simulink model "quad_LQRwithIntegrators_sim"  (R2020a)
settings: Solver=ode4  StartTime=0.0  StopTime=5  FixedStep=0.001  RelTol=1e-3
values from neighbouring files (symbols this model uses):
  L = 0.2    [anim_2Dquad.m]    (also in anim_2Dquad_intercept.m)
undefined symbols (not defined in the file or in its folder): g, I, K_aug, m
settings Model: Creator=Amir  LastModifiedBy=alex
settings DataIOCC: ReturnWorkspaceOutputs=off
settings DebuggingCC: ArithmeticOperatorsInVariantConditions=warning
settings SFSimCC: CustomCodeUndefinedFunction=UseInterfaceOnly

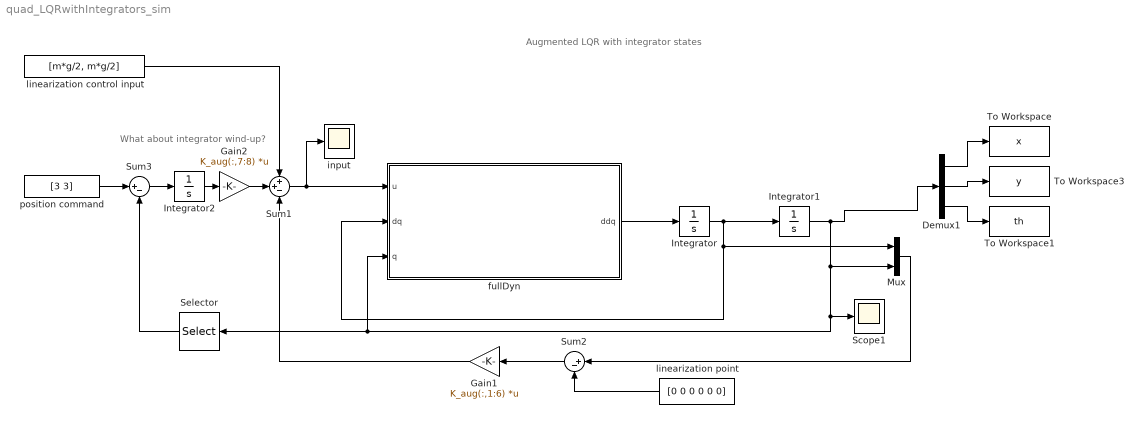
== system quad_LQRwithIntegrators_sim ==
  note: Augmented LQR with integrator states
  note: What about integrator wind-up?
  Demux1 : Demux  Outputs=3
  Gain1 : Gain  Gain=K_aug(:,1:6)  Multiplication=Matrix(K*u)
  Gain2 : Gain  Gain=K_aug(:,7:8)  Multiplication=Matrix(K*u)
  Integrator : Integrator  InitialCondition=[0 0 0]
  Integrator1 : Integrator  InitialCondition=[0, 0, 0]
  Integrator2 : Integrator
  Mux : Mux  Inputs=2
  Scope1 : Scope
  Selector : Selector  InputPortWidth=3  IndexOptions=Index vector (dialog)  Indices=[1 2]  OutputSizes=1
  Sum1 : Sum  Inputs=++-
  Sum2 : Sum  Inputs=|+-
  Sum3 : Sum  Inputs=|+-
  To Workspace : ToWorkspace  VariableName=x  SaveFormat=Structure With Time  SampleTime=0.01
  To Workspace1 : ToWorkspace  VariableName=th  SaveFormat=Structure With Time  SampleTime=0.01
  To Workspace3 : ToWorkspace  VariableName=y  SaveFormat=Structure With Time  SampleTime=0.01
  fullDyn : MATLAB Function  TreatAsAtomicUnit=on
  input : Scope
  linearization control input : Constant  Value=[m*g/2, m*g/2]
  linearization point : Constant  Value=[0 0 0 0 0 0]
  position command : Constant  Value=[3 3]
  wires:
  fullDyn/1(ddq) -> Integrator/1
  Integrator/1 -> Integrator1/1, Mux/1, fullDyn/2(dq)
  Integrator1/1 -> Demux1/1, Mux/2, Scope1/1, fullDyn/3(q), Selector/1
  Sum1/1 -> input/1, fullDyn/1(u)
  Sum2/1 -> Gain1/1
  linearization point/1 -> Sum2/2
  Mux/1 -> Sum2/1
  linearization control input/1 -> Sum1/1
  Gain1/1 -> Sum1/3
  Integrator2/1 -> Gain2/1
  Gain2/1 -> Sum1/2
  Sum3/1 -> Integrator2/1
  position command/1 -> Sum3/1
  Selector/1 -> Sum3/2
  Demux1/1 -> To Workspace/1
  Demux1/2 -> To Workspace3/1
  Demux1/3 -> To Workspace1/1

== matlab function quad_LQRwithIntegrators_sim/fullDyn ==
  data: u input; ddq output; dq input; q input; m parameter; I parameter; L parameter; g parameter
function ddq = fullDyn(u,dq,q, m, I, L, g)
%#codegen

%    This function was generated by the Symbolic Math Toolbox version 8.2.
%    23-Apr-2019 00:12:18
% m = 10;
% L = 0.5;
% I = 0.2083; %MOI of a thin rod
% g = 9.81;

F1 = u(1);
F2 = u(2);

x = q(1);
y = q(2);
th = q(3);

dx = dq(1);
dy = dq(2);
dth = dq(3);

t2 = cos(th);
t3 = 1.0./m;
ddq = [-t3.*sin(th).*(F1+F2);t3.*(F1.*t2+F2.*t2-g.*m);(L.*(F1-F2))./(I.*2.0)];
